simulink model "block_diagram_reduction_simulink"  (R2026a)
settings: Solver=VariableStepAuto  StopTime=2
settings Model: Creator=PC-Admin  LastModifiedBy=PC-Admin

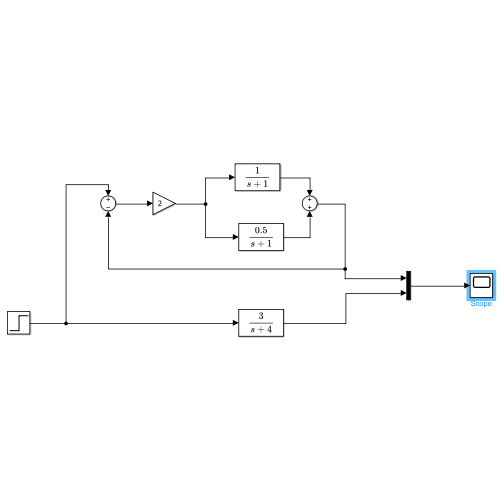
[thumbnail: Simulink's stored preview of the top-level diagram]
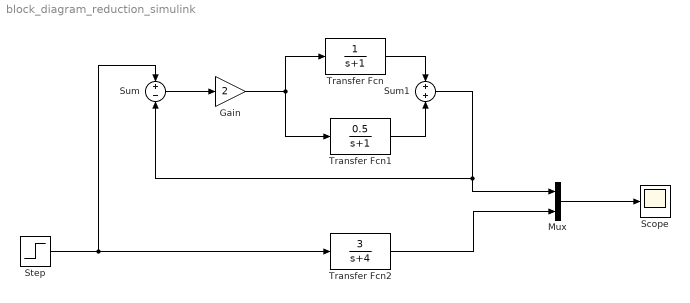
== system block_diagram_reduction_simulink ==
  Gain : Gain  Gain=2
  Mux : Mux  Inputs=2
  Scope : Scope
      settings: ActiveDisplayYMinimum=-0.52017846970096093  ActiveDisplayYMaximum=1.0538965883862175
  Step : Step  SampleTime=0
  Sum : Sum  Inputs=+-
  Sum1 : Sum
  Transfer Fcn : TransferFcn  Denominator=[1 1]
  Transfer Fcn1 : TransferFcn  Numerator=[0.5]  Denominator=[1 1]
  Transfer Fcn2 : TransferFcn  Numerator=[3]  Denominator=[1 4]
  wires:
  Step/1 -> Transfer Fcn2/1, Sum/1
  Sum/1 -> Gain/1
  Gain/1 -> Transfer Fcn1/1, Transfer Fcn/1
  Transfer Fcn/1 -> Sum1/1
  Transfer Fcn1/1 -> Sum1/2
  Sum1/1 -> Mux/1, Sum/2
  Transfer Fcn2/1 -> Mux/2
  Mux/1 -> Scope/1
